simulink model "Tones_2"  (R2022a)
settings: Solver=FixedStepAuto  StartTime=0.0  StopTime=inf  FixedStep=Ts  RelTol=1e-3  EnableMultiTasking=on
InitFcn:
  | n = 4; %order n
  | fs = 5000;
  | Ts =1/fs;
  | %% %%%%%%%%%%%% allow 80 and 200 Hz %%%%%%%%%%%%%%
  | Wn = [10 400]
  | Wn = Wn/(fs/2); %cutoff frequency
  | [b2,a2] = butter(n,Wn,'bandpass');
  | % bode(tf(b2,a2,1/fs))
  | 
  | %% %%%%%%%%%%%% allow 500 and 800 Hz %%%%%%%%%%%%%%
  | Wn = [300 1000];
  | Wn = Wn/(fs/2); %cutoff frequency
  | [b3,a3] = butter(n,Wn,'bandpass');
  | % bode(tf(b3,a3,1/fs));
  | 
  | %% %%%%%%%%%%%% allow none  %%%%%%%%%%%%%%
  | n=4;
  | Wn = [130 600];
  | Wn = Wn/(fs/2); %cutoff frequency
  | [b4,a4] = butter(n,Wn,'stop');
  | % bode(tf(b4,a4,1/fs));
  | 
  |  %%%%%%%%%%%% allow none  %%%%%%%%%%%%%%
  |  n=4;
  | Wn = 130;
  | Wn = Wn/(fs/2); %cutoff frequency
  | [b4l,a4l] = butter(n,Wn,'low');
  | Wn = 600;
  | Wn = Wn/(fs/2); %cutoff frequency
  | [b4h,a4h] = butter(n,Wn,'high');
  | fl = tf(b4l,a4l,1/fs)*tf(b4h,a4h,1/fs);
  | % bode(fl);
undefined symbols (not defined in the file): a2, a3, a4h, a4l, b2, b3, b4h, b4l, bias
libraries: arduinolib x3
settings Model: ExtModeTrigDuration=2  Creator=mshafiqu  LastModifiedBy=Kostas Tsakalis
settings SolverCC: AlgebraicLoopSolver=TrustRegion
settings DataIOCC: LimitDataPoints=on  ReturnWorkspaceOutputs=off
settings OptimizationCC: LifeSpan=1  MaxStackSize=64  EfficientTunableParamExpr=on
settings DebuggingCC: UnconnectedInputMsg=warning  UnconnectedOutputMsg=warning  UnconnectedLineMsg=warning  AllowSymbolicDim=off  SFUnexpectedBacktrackingDiag=warning  SFNoUnconditionalDefaultTransitionDiag=warning  SFExecutionAtInitializationDiag=none  SFMachineParentedDataDiag=warning  ArithmeticOperatorsInVariantConditions=warning
settings HardwareCC: ProdBitPerPointer=32  ProdBitPerSizeT=32  ProdBitPerPtrDiffT=32  ProdLargestAtomicInteger=Long  ProdLargestAtomicFloat=Double  ProdWordSize=32  ProdHWDeviceType=ARM Compatible->ARM Cortex  UseEmbeddedCoderFeatures=off  UseSimulinkCoderFeatures=off
settings ModelReferenceCC: PropagateSignalLabelsOutOfModel=off
settings SFSimCC: SimUseLocalCustomCode=off  MATLABDynamicMemAlloc=off  CustomCodeUndefinedFunction=UseInterfaceOnly
settings RTWCC: SystemTargetFile=ert.tlc  HardwareBoard=Arduino Due  TemplateMakefile=ert_default_tmf  RTWUseLocalCustomCode=off  Toolchain=Arduino ARM  BuildConfiguration=Faster Runs
settings CodeAppCC: IgnoreCustomStorageClasses=off  MangleLength=10  StateflowObjectComments=on
settings ERTTargetCC: MultiwordLength=2048  SupportContinuousTime=on  SupportNonInlinedSFcns=on  SupportVariableSizeSignals=on  ConvertIfToSwitch=off  SuppressUnreachableDefaultCases=off
settings ConfigComp: CovMetricSettings=dw  CovSaveCumulativeToWorkspaceVar=on  CovSaveSingleToWorkspaceVar=on  CovExternalEMLEnable=off

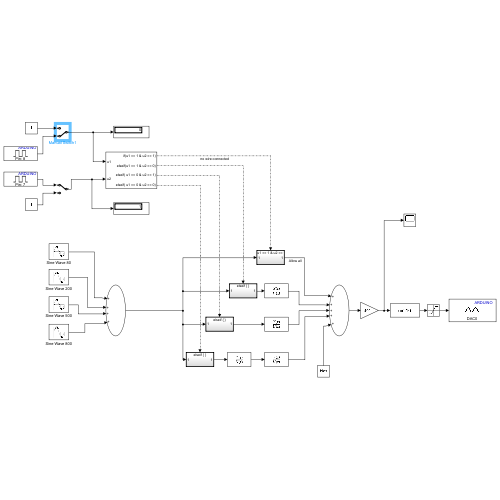
[thumbnail: Simulink's stored preview of the top-level diagram]
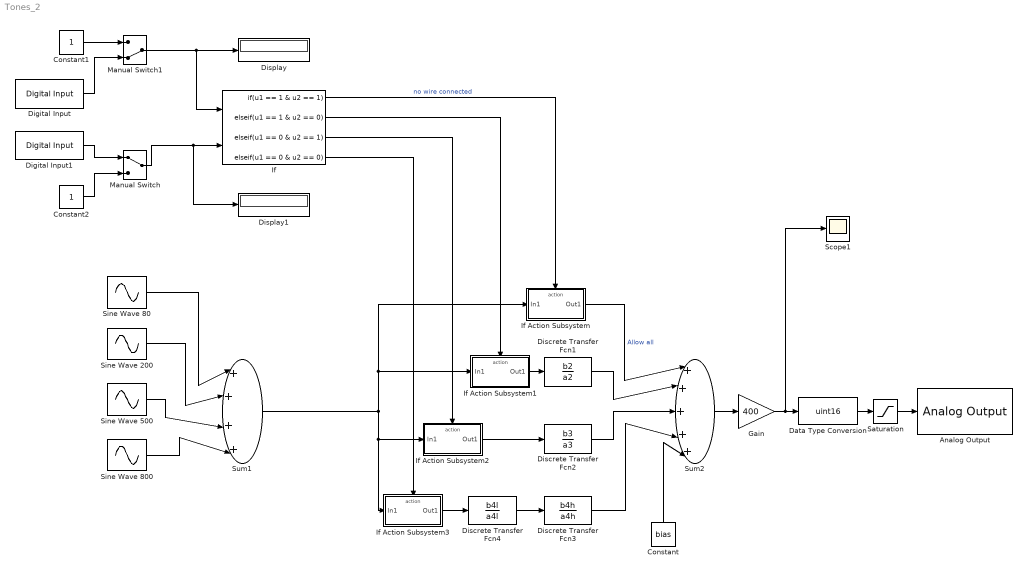
== system Tones_2 ==
  Analog Output : arduinolib/Analog Output  DACpin=DAC0  blockPlatform=arduino
      settings: SourceProductBaseCode=ARDUINO
  Constant : Constant  Value=bias  SampleTime=Ts
  Constant1 : Constant  SampleTime=Ts
  Constant2 : Constant  SampleTime=Ts
  Data Type Conversion : DataTypeConversion  OutDataTypeStr=uint16  SaturateOnIntegerOverflow=off  RndMeth=Floor
  Digital Input : arduinolib/Digital Input  pinNumber=8  mode=Default  Direction=input  SampleTime=Ts  blockPlatform=arduino
  Digital Input1 : arduinolib/Digital Input  pinNumber=7  mode=Default  Direction=input  SampleTime=Ts  blockPlatform=arduino
  Discrete Transfer Fcn1 : DiscreteTransferFcn  Numerator=b2  Denominator=a2  SampleTime=Ts
  Discrete Transfer Fcn2 : DiscreteTransferFcn  Numerator=b3  Denominator=a3  SampleTime=Ts
  Discrete Transfer Fcn3 : DiscreteTransferFcn  Numerator=b4h  Denominator=a4h  SampleTime=Ts
  Discrete Transfer Fcn4 : DiscreteTransferFcn  Numerator=b4l  Denominator=a4l  SampleTime=Ts
  Display : Display
  Display1 : Display
  Gain : Gain  Gain=400
  If : If  NumInputs=2  IfExpression=u1 == 1 & u2 == 1  ElseIfExpressions=u1 == 1 & u2 == 0, u1 == 0 & u2 == 1, u1 == 0 & u2 == 0  ShowElse=off
  If Action Subsystem : Subsystem  TreatAsAtomicUnit=on
  If Action Subsystem1 : Subsystem  TreatAsAtomicUnit=on
  If Action Subsystem2 : Subsystem  TreatAsAtomicUnit=on
  If Action Subsystem3 : Subsystem  TreatAsAtomicUnit=on
  Manual Switch : ManualSwitch
  Manual Switch1 : ManualSwitch  CurrentSetting=0
  Saturation : Saturate  UpperLimit=3000  LowerLimit=100
  Scope1 : Scope
  Sine Wave 200 : Sin  Amplitude=0.5  Frequency=2*pi*200  Samples=125  SampleTime=Ts
  Sine Wave 500 : Sin  Amplitude=0.5  Frequency=2*pi*500  Samples=125  SampleTime=Ts
  Sine Wave 80 : Sin  Amplitude=0.5  Frequency=2*pi*80  Samples=125  SampleTime=Ts
  Sine Wave 800 : Sin  Amplitude=0.5  Frequency=2*pi*800  Samples=125  SampleTime=Ts
  Sum1 : Sum  Inputs=|++++|
  Sum2 : Sum  Inputs=|+++++|
  wires:
  Data Type Conversion/1 -> Saturation/1
  Sine Wave 80/1 -> Sum1/1
  Sine Wave 200/1 -> Sum1/2
  Constant/1 -> Sum2/5
  Sine Wave 500/1 -> Sum1/3
  Sine Wave 800/1 -> Sum1/4
  Saturation/1 -> Analog Output/1
  Sum1/1 -> If Action Subsystem3/1(In1), If Action Subsystem2/1(In1), If Action Subsystem1/1(In1), If Action Subsystem/1(In1)
  Manual Switch1/1 -> If/1, Display/1
  Manual Switch/1 -> Display1/1, If/2
  If Action Subsystem1/1(Out1) -> Discrete Transfer Fcn1/1
  If Action Subsystem2/1(Out1) -> Discrete Transfer Fcn2/1
  If/1 -> If Action Subsystem/Action  "no wire connected"
  If/2 -> If Action Subsystem1/Action
  If/3 -> If Action Subsystem2/Action
  If/4 -> If Action Subsystem3/Action
  Discrete Transfer Fcn3/1 -> Sum2/4
  If Action Subsystem/1(Out1) -> Sum2/1  "Allow all"
  Discrete Transfer Fcn1/1 -> Sum2/2
  Discrete Transfer Fcn2/1 -> Sum2/3
  Gain/1 -> Scope1/1, Data Type Conversion/1
  Sum2/1 -> Gain/1
  Constant2/1 -> Manual Switch/2
  Constant1/1 -> Manual Switch1/1
  Digital Input/1 -> Manual Switch1/2
  Digital Input1/1 -> Manual Switch/1
  If Action Subsystem3/1(Out1) -> Discrete Transfer Fcn4/1
  Discrete Transfer Fcn4/1 -> Discrete Transfer Fcn3/1

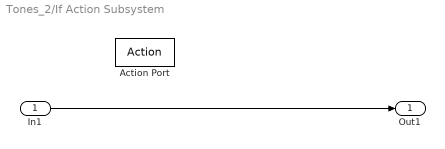
== system Tones_2/If Action Subsystem ==
  In1 : Inport
  Action Port : ActionPort  InitializeStates=reset  ActionPortLabel=if(u1 == 1 & u2 == 1)
  Out1 : Outport  OutputWhenDisabled=reset  InitialOutput=0
  wires:
  In1/1 -> Out1/1

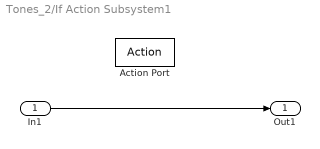
== system Tones_2/If Action Subsystem1 ==
  In1 : Inport
  Action Port : ActionPort  InitializeStates=reset  ActionPortLabel=elseif(u1 == 1 & u2 == 0)
  Out1 : Outport  OutputWhenDisabled=reset  InitialOutput=0
  wires:
  In1/1 -> Out1/1

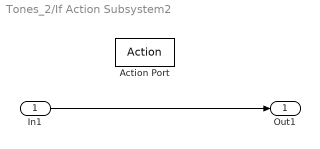
== system Tones_2/If Action Subsystem2 ==
  In1 : Inport
  Action Port : ActionPort  InitializeStates=reset  ActionPortLabel=elseif( u1 == 0 & u2 == 1)
  Out1 : Outport  OutputWhenDisabled=reset  InitialOutput=0
  wires:
  In1/1 -> Out1/1

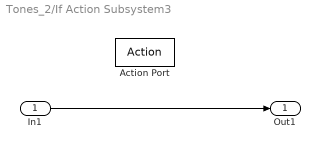
== system Tones_2/If Action Subsystem3 ==
  In1 : Inport
  Action Port : ActionPort  InitializeStates=reset  ActionPortLabel=elseif( u1 == 0 & u2 == 0)
  Out1 : Outport  OutputWhenDisabled=reset  InitialOutput=0
  wires:
  In1/1 -> Out1/1
